simulink model "slb_vector"  (R2015b)
settings: Solver=FixedStepDiscrete  SolverMode=SingleTasking  StartTime=0.0  StopTime=10  RelTol=1e-3
CloseFcn:
  | rtwprivate ssgencode ModelCloseRequest Hysteresis_test1
settings Model: Creator=at-mt  LastModifiedBy=amatsumo
settings DataIOCC: SaveFormat=Array  SignalLoggingSaveFormat=ModelDataLogs  SaveOutput=off  SignalLogging=off  SaveTime=off
settings OptimizationCC: BlockReduction=off  ConditionallyExecuteInputs=off  DefaultParameterBehavior=Inlined  ExpressionDepthLimit=2147483647
settings DebuggingCC: AlgebraicLoopMsg=error  UnderspecifiedInitializationDetection=Classic  MergeDetectMultiDrivingBlocksExec=none  SolverPrmCheckMsg=warning  SingleTaskRateTransMsg=error  FcnCallInpInsideContextMsg=UseLocalSettings  StateNameClashWarn=warning
settings HardwareCC: ProdBitPerPointer=32  ProdLargestAtomicFloat=None  ProdIntDivRoundTo=Undefined  ProdEndianess=Unspecified  ProdWordSize=32  ProdHWDeviceType=ASIC/FPGA->ASIC/FPGA  ProdEqTarget=off
settings GRTTargetCC: GeneratePreprocessorConditionals=Disable all  CombineOutputUpdateFcns=off  GRTInterface=on
settings ConfigComp: CovModelRefEnable=Off  CovSFcnEnable=off

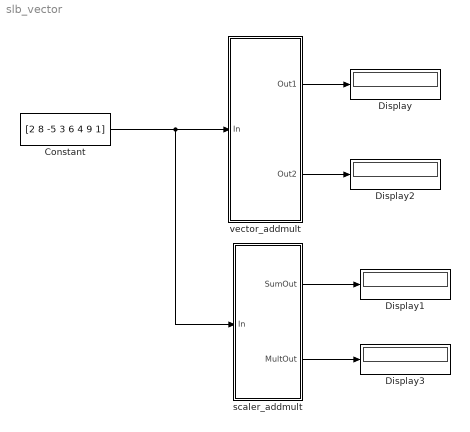
== system slb_vector ==
  Constant : Constant  Value=[2 8 -5 3 6 4 9 1]  OutDataTypeStr=int8  SampleTime=1
  Display{,1..3} (4 alike) : Display
  scaler_addmult : Subsystem
  vector_addmult : Subsystem
  wires:
  scaler_addmult/1(SumOut) -> Display1/1
  scaler_addmult/2(MultOut) -> Display3/1
  vector_addmult/2(Out2) -> Display2/1
  vector_addmult/1(Out1) -> Display/1
  Constant/1 -> vector_addmult/1(In), scaler_addmult/1(In)

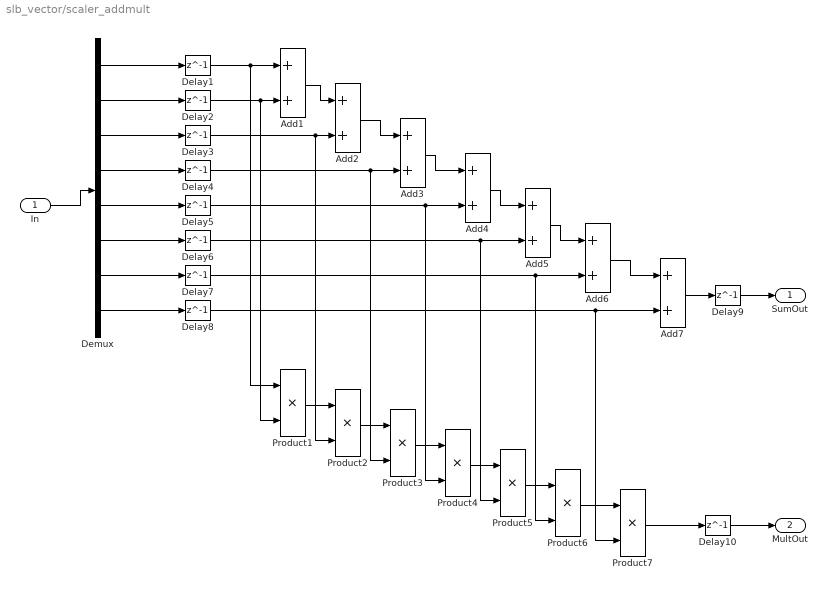
== system slb_vector/scaler_addmult ==
  In : Inport
  Add{1..7} (7 alike) : Sum
  Delay{1..10} (10 alike) : Delay  DelayLength=1  InputProcessing=Inherited
  Demux : Demux  Outputs=8
  Product{1..7} (7 alike) : Product  RndMeth=Zero
  SumOut : Outport
  MultOut : Outport  Port=2
  wires:
  Delay10/1 -> MultOut/1
  Delay9/1 -> SumOut/1
  In/1 -> Demux/1
  Demux/1 -> Delay1/1
  Demux/2 -> Delay2/1
  Demux/3 -> Delay3/1
  Demux/4 -> Delay4/1
  Demux/5 -> Delay5/1
  Demux/6 -> Delay6/1
  Demux/7 -> Delay7/1
  Demux/8 -> Delay8/1
  Delay1/1 -> Add1/1, Product1/1
  Delay2/1 -> Add1/2, Product1/2
  Add1/1 -> Add2/1
  Delay3/1 -> Add2/2, Product2/2
  Delay4/1 -> Add3/2, Product3/2
  Add2/1 -> Add3/1
  Delay5/1 -> Add4/2, Product4/2
  Add3/1 -> Add4/1
  Delay6/1 -> Add5/2, Product5/2
  Add4/1 -> Add5/1
  Delay7/1 -> Add6/2, Product6/2
  Add5/1 -> Add6/1
  Delay8/1 -> Add7/2, Product7/2
  Add6/1 -> Add7/1
  Add7/1 -> Delay9/1
  Product1/1 -> Product2/1
  Product2/1 -> Product3/1
  Product3/1 -> Product4/1
  Product4/1 -> Product5/1
  Product5/1 -> Product6/1
  Product6/1 -> Product7/1
  Product7/1 -> Delay10/1

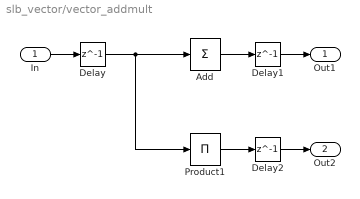
== system slb_vector/vector_addmult ==
  In : Inport
  Add : Sum  Inputs=+  OutDataTypeStr=fixdt(1,15,0)  RndMeth=Nearest
  Delay : Delay  DelayLength=1
  Delay1 : Delay  DelayLength=1
  Delay2 : Delay  DelayLength=1
  Product1 : Product  Inputs=1  OutDataTypeStr=fixdt(1,64,0)  RndMeth=Nearest
  Out1 : Outport
  Out2 : Outport  Port=2
  wires:
  Delay/1 -> Product1/1, Add/1
  Add/1 -> Delay1/1
  Product1/1 -> Delay2/1
  Delay1/1 -> Out1/1
  Delay2/1 -> Out2/1
  In/1 -> Delay/1
